simulink model "Windgeschwindigkeitsgenerator"  (R2022b)
settings: Solver=ode4  StartTime=0.0  StopTime=Tmax  FixedStep=dT  RelTol=1e-3  EnableMultiTasking=on
values from neighbouring files (symbols this model uses):
  dT = 0.01    [Windgenerator.m]
undefined symbols (not defined in the file or in its folder): Param_Wind
settings Model: Creator=georg  LastModifiedBy=Aaron
settings SolverCC: AlgebraicLoopSolver=TrustRegion
settings DataIOCC: LimitDataPoints=on  SaveFormat=Array
settings OptimizationCC: DefaultParameterBehavior=Inlined  ExpressionDepthLimit=2147483647  LifeSpan=inf
settings DebuggingCC: UnderspecifiedInitializationDetection=Classic  MergeDetectMultiDrivingBlocksExec=none  SolverPrmCheckMsg=warning  FcnCallInpInsideContextMsg=warning  UnconnectedInputMsg=warning  UnconnectedOutputMsg=warning  UnconnectedLineMsg=warning  StateNameClashWarn=warning  SFUnexpectedBacktrackingDiag=warning  SFNoUnconditionalDefaultTransitionDiag=warning  SFMachineParentedDataDiag=warning  ArithmeticOperatorsInVariantConditions=warning
settings HardwareCC: ProdBitPerPointer=32  ProdBitPerSizeT=32  ProdBitPerPtrDiffT=32  ProdLargestAtomicFloat=None  ProdIntDivRoundTo=Undefined  ProdEndianess=Unspecified  ProdWordSize=32  ProdHWDeviceType=32-bit Generic
settings ModelReferenceCC: EnableRefExpFcnMdlSchedulingChecks=on  PropagateSignalLabelsOutOfModel=off
settings SFSimCC: SimUseLocalCustomCode=off  CustomCodeUndefinedFunction=UseInterfaceOnly
settings RTWCC: RTWUseLocalCustomCode=off
settings CodeAppCC: StateflowObjectComments=on
settings GRTTargetCC: TargetLangStandard=C89/C90 (ANSI)  CombineOutputUpdateFcns=off  GRTInterface=on
settings ConfigComp: CovMetricSettings=dw  CovSaveCumulativeToWorkspaceVar=on  CovSaveSingleToWorkspaceVar=on  CovExternalEMLEnable=off

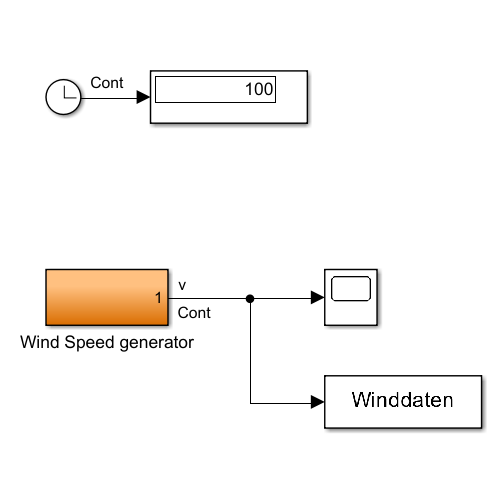
[thumbnail: Simulink's stored preview of the top-level diagram]
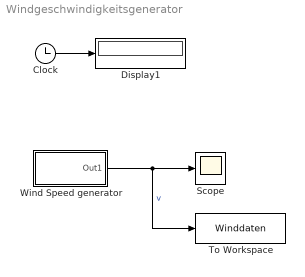
== system Windgeschwindigkeitsgenerator ==
  Clock : Clock
  Display1 : Display
  Scope : Scope
  To Workspace : ToWorkspace  VariableName=Winddaten  SaveFormat=Structure With Time  SampleTime=-1
  Wind Speed generator : Subsystem
  wires:
  Clock/1 -> Display1/1
  Wind Speed generator/1(Out1) -> To Workspace/1, Scope/1  "v"

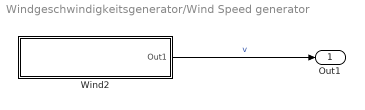
== system Windgeschwindigkeitsgenerator/Wind Speed generator ==
  Wind2 : Subsystem
  Out1 : Outport
  wires:
  Wind2/1(Out1) -> Out1/1  "v"

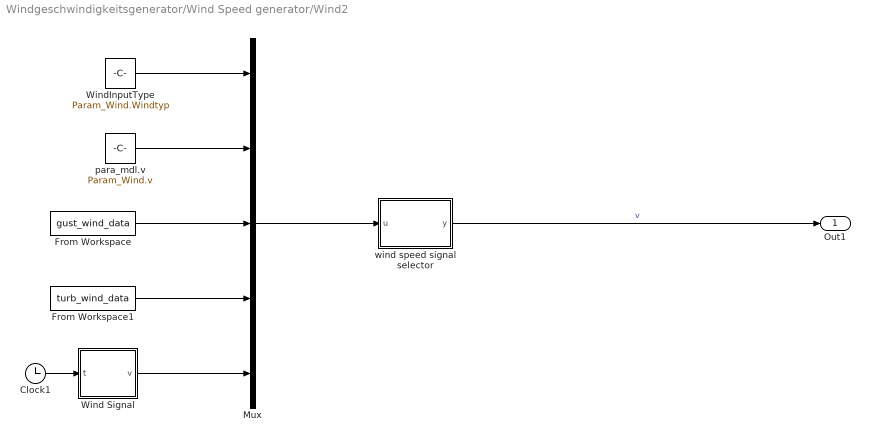
== system Windgeschwindigkeitsgenerator/Wind Speed generator/Wind2 ==
  Clock1 : Clock
  From Workspace : FromWorkspace  VariableName=gust_wind_data  SampleTime=dT  OutputAfterFinalValue=Holding final value
  From Workspace1 : FromWorkspace  VariableName=turb_wind_data  SampleTime=dT  OutputAfterFinalValue=Holding final value
  Mux : Mux  Inputs=5
  Wind Signal : MATLAB Function  TreatAsAtomicUnit=on
  WindInputType : Constant  Value=Param_Wind.Windtyp
  para_mdl.v : Constant  Value=Param_Wind.v
  wind speed signal selector : MATLAB Function  TreatAsAtomicUnit=on
  Out1 : Outport
  wires:
  Wind Signal/1(v) -> Mux/5
  Clock1/1 -> Wind Signal/1(t)
  Mux/1 -> wind speed signal selector/1(u)
  wind speed signal selector/1(y) -> Out1/1  "v"
  WindInputType/1 -> Mux/1
  para_mdl.v/1 -> Mux/2
  From Workspace/1 -> Mux/3
  From Workspace1/1 -> Mux/4

== matlab function Windgeschwindigkeitsgenerator/Wind Speed generator/Wind2/Wind Signal ==
  data: t input; v output
function v = step(t)

t_step_1    = 10;
t_step_2    = 30;
v1          = 4;  
delta_v     = 3;
%delta_v2    =   9 - delta_v - v1;   % nur Teillast
delta_v2    = 25 - delta_v - v1;   % Teillast -> Vollast

if t <= t_step_1
    v = v1;
elseif t <= t_step_2
    v = v1 + delta_v;
else
    v = v1 + delta_v + delta_v2;
end

== matlab function Windgeschwindigkeitsgenerator/Wind Speed generator/Wind2/wind speed signal selector ==
  data: u input; y output
function y = fcn(u)

i = u(1);

y = u(i+1);
